simulink model "can_decoder"  (R2025a)
settings: configuration reference "AMCBLDC_Configuration" (kept outside this file)
undefined symbols (not defined in the file): CAN_ID_AMC, CAN_VOLT_REF_GAIN, CAN_VOLT_REF_SHIFT
settings Model: DataDictionary=amcbldc.sldd  Creator=upattacini  LastModifiedBy=rpumpo
settings ConfigSetRef: SourceName=AMCBLDC_Configuration

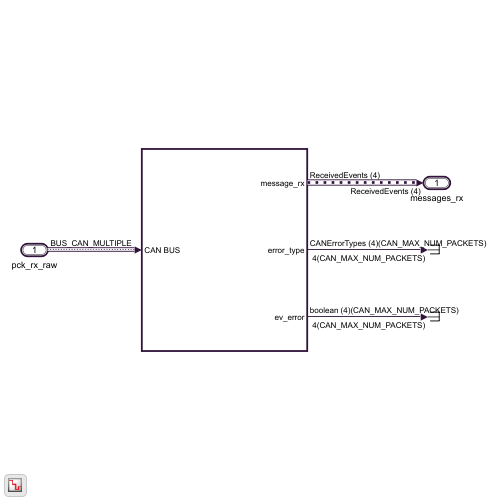
[thumbnail: Simulink's stored preview of the top-level diagram]
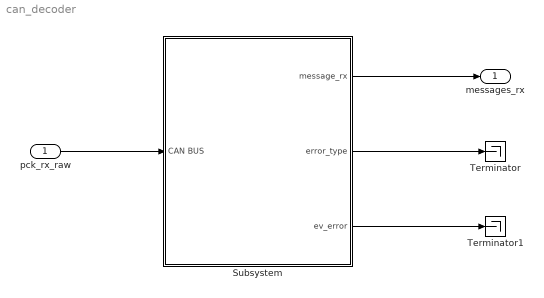
== system can_decoder ==
  pck_rx_raw : Inport  OutDataTypeStr=Bus: BUS_CAN_MULTIPLE  BusOutputAsStruct=on
  Subsystem : Subsystem
  Terminator : Terminator
  Terminator1 : Terminator
  messages_rx : Outport  OutDataTypeStr=Bus: ReceivedEvents  BusOutputAsStruct=on
  wires:
  pck_rx_raw/1 -> Subsystem/1(CAN BUS)
  Subsystem/1(message_rx) -> messages_rx/1
  Subsystem/2(error_type) -> Terminator/1
  Subsystem/3(ev_error) -> Terminator1/1

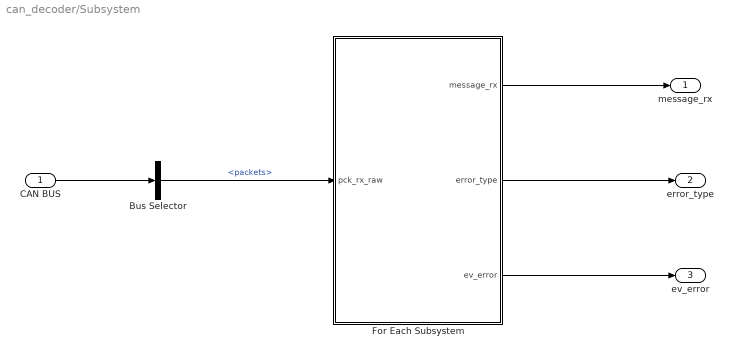
== system can_decoder/Subsystem ==
  CAN BUS : Inport
  Bus Selector : BusSelector  OutputSignals=packets
  For Each Subsystem : Subsystem  TreatAsAtomicUnit=on
  message_rx : Outport  PortDimensions=4
  error_type : Outport  Port=2
  ev_error : Outport  Port=3
  wires:
  Bus Selector/1 -> For Each Subsystem/1(pck_rx_raw)  "<packets>"
  CAN BUS/1 -> Bus Selector/1
  For Each Subsystem/3(ev_error) -> ev_error/1
  For Each Subsystem/1(message_rx) -> message_rx/1
  For Each Subsystem/2(error_type) -> error_type/1

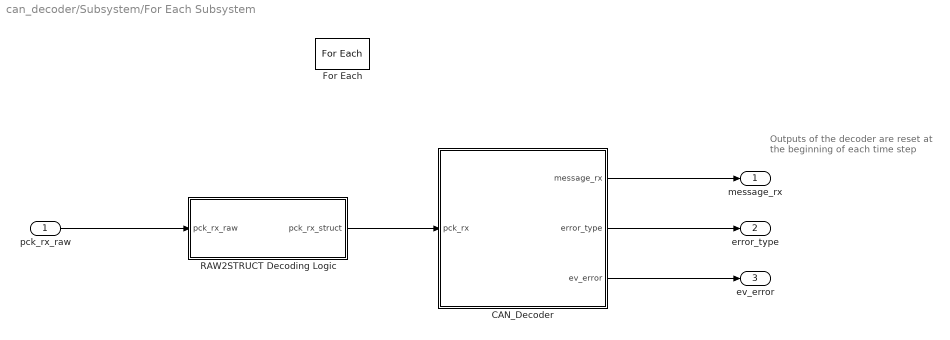
== system can_decoder/Subsystem/For Each Subsystem ==
  note: Outputs of the decoder are reset at
      | the beginning of each time step
  pck_rx_raw : Inport  Partition=on  PartitionDimension=1  PartitionWidth=1  PartitionOffset=0
  CAN_Decoder : Subsystem  TreatAsAtomicUnit=on
  For Each : ForEach  DisableCoverage=on  SpecifiedNumIters=CAN_MAX_NUM_PACKETS
  RAW2STRUCT Decoding Logic : MATLAB Function  TreatAsAtomicUnit=on
  message_rx : Outport  OutDataTypeStr=Bus: ReceivedEvents  ConcatenationDimension=1
  error_type : Outport  Port=2  ConcatenationDimension=1
  ev_error : Outport  Port=3  ConcatenationDimension=1
  wires:
  CAN_Decoder/3(ev_error) -> ev_error/1
  RAW2STRUCT Decoding Logic/1(pck_rx_struct) -> CAN_Decoder/1(pck_rx)
  CAN_Decoder/1(message_rx) -> message_rx/1
  pck_rx_raw/1 -> RAW2STRUCT Decoding Logic/1(pck_rx_raw)
  CAN_Decoder/2(error_type) -> error_type/1

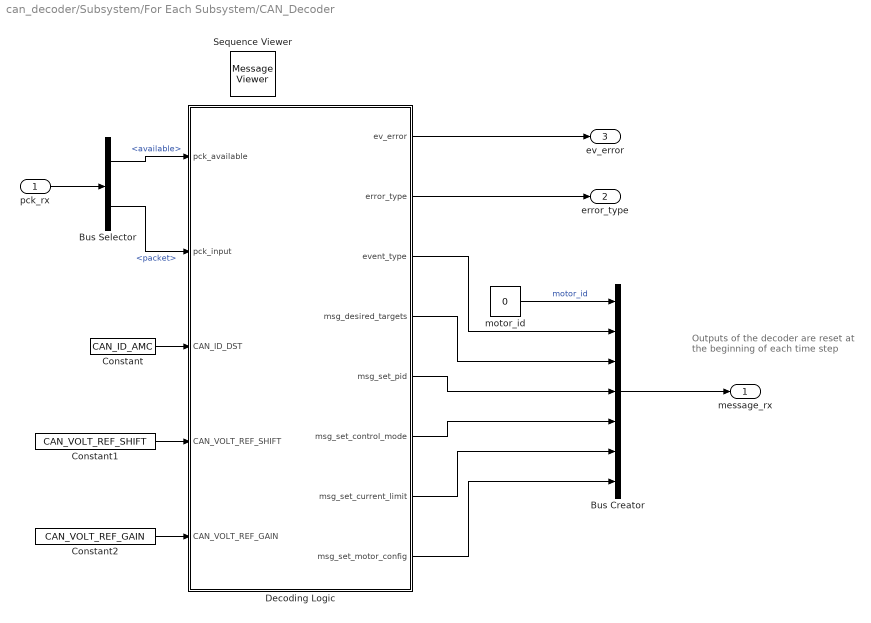
== system can_decoder/Subsystem/For Each Subsystem/CAN_Decoder ==
  note: Outputs of the decoder are reset at
      | the beginning of each time step
  pck_rx : Inport  OutDataTypeStr=Bus: BUS_CAN_RX
  Bus Creator : BusCreator  Inputs=7  OutDataTypeStr=Bus: ReceivedEvents  NonVirtualBus=on
      settings: InheritFromInputs=off
  Bus Selector : BusSelector  OutputSignals=available,packet
  Constant : Constant  Value=CAN_ID_AMC  OutDataTypeStr=uint8
  Constant1 : Constant  Value=CAN_VOLT_REF_SHIFT  OutDataTypeStr=uint8
  Constant2 : Constant  Value=CAN_VOLT_REF_GAIN  OutDataTypeStr=single
  Decoding Logic : Stateflow chart  TreatAsAtomicUnit=on
      settings: PortSchema="{\"entries\":[{\"content\":{\"sides\":[{\"content\":{\"connectorIds\":[\"In1\",\"In2\",\"In3\",\"In4\",\"In5\"]},\"type\":\"ConnectorPlacement.EquallySpacedRectSide\",\"uuid\":\"bb5ffdcb-390f-4d7b-9f99-b75bae8a05ad\"},{\"content\":{\"connectorIds\":[\"Out8\",\"Out6\",\"Out7\",\"Out3\",\"Out4\",\"Out1\",\"Out2\",\"Out5\"],\"side\":\"RIGHT\"},\"type\":\"ConnectorPlacement.EquallySpacedRectSide\",\"uuid\":\"3ba90815-a3e4-4cd4-b64a-5c95e1f5d631\"},{\"content\":{\"side\":\"TOP\"},\"type\":\"ConnectorPlacement.EquallySpacedRectSide\",\"uuid\":\"c9c9b262-1031-4ca9-8b93-619604387376\"}]},\"type\":\"ConnectorPlacement.EquallySpacedConnector\",\"uuid\":\"025015ea-955c-40a8-a93e-b34368e10f0a\"}],\"packageUris\":[\"http://schema.mathworks.com/mf0/Connector/R2020b\"],\"version\":\"1.0\"}"
  Sequence Viewer : MessageViewer
  motor_id : Constant  Value=0  OutDataTypeStr=uint8
  message_rx : Outport  OutDataTypeStr=Bus: ReceivedEvents
  error_type : Outport  Port=2
  ev_error : Outport  Port=3
  wires:
  Constant/1 -> Decoding Logic/3(CAN_ID_DST)
  pck_rx/1 -> Bus Selector/1
  Bus Selector/1 -> Decoding Logic/1(pck_available)  "<available>"
  Bus Selector/2 -> Decoding Logic/2(pck_input)  "<packet>"
  Constant1/1 -> Decoding Logic/4(CAN_VOLT_REF_SHIFT)
  Constant2/1 -> Decoding Logic/5(CAN_VOLT_REF_GAIN)
  Decoding Logic/8(ev_error) -> ev_error/1
  Decoding Logic/6(error_type) -> error_type/1
  Bus Creator/1 -> message_rx/1
  Decoding Logic/7(event_type) -> Bus Creator/2
  Decoding Logic/3(msg_desired_targets) -> Bus Creator/3
  Decoding Logic/4(msg_set_pid) -> Bus Creator/4
  Decoding Logic/1(msg_set_control_mode) -> Bus Creator/5
  Decoding Logic/2(msg_set_current_limit) -> Bus Creator/6
  Decoding Logic/5(msg_set_motor_config) -> Bus Creator/7
  motor_id/1 -> Bus Creator/1  "motor_id"

== stateflow chart can_decoder/Subsystem/For Each Subsystem/CAN_Decoder/Decoding Logic ==
  settings: initializeOutput=1  description=This state chart is responsible for decoding incoming CAN packets.
  state ErrorHandler [parallel]
    settings: executionOrder=2
    state Home
      entry:
      cmd_processed = 0;
      exit:
      ev_async = false;
    state Event_Error
      entry:
      ev_async = true;
    (default) -> ErrorHandler.Home
    (junction 111) -> ErrorHandler.Home [order 2] : {error_type = CANErrorTypes.No_Error;}
    (junction 111) -> ErrorHandler.Home [order 1] : [cmd_processed > 1]
        | {error_type = CANErrorTypes.Packet_MultiFunctionsDetected;
        | send(ev_error);}
    ErrorHandler.Home -> ErrorHandler.Home [order 4] : [ev_async]
    (junction 109) -> ErrorHandler.Home [order 1] : [pck_available && (cmd_processed == 0)]
        | {error_type = CANErrorTypes.Packet_Unrecognized;
        | send(ev_error);}
    Event_Error -> ErrorHandler.Home
    ErrorHandler.Home -> Event_Error [order 1] : ev_error_pck_not4us
        | {error_type = CANErrorTypes.Packet_Not4Us;
        | send(ev_error);}
    ErrorHandler.Home -> Event_Error [order 2] : ev_error_pck_malformed
        | {error_type = CANErrorTypes.Packet_Malformed;
        | send(ev_error);}
    ErrorHandler.Home -> Event_Error [order 3] : ev_error_mode_unrecognized
        | {error_type = CANErrorTypes.Mode_Unrecognized;
        | send(ev_error);}
    ErrorHandler.Home -> (junction 109) [order 5]
    (junction 109) -> (junction 111) [order 2]
  state CANParser [parallel]
    settings: executionOrder=1
    state Home
    state SetCommand [function]
      state r = isPayloadValid(expected_size) [function]
        (default) -> (junction 402) : {r = true;}
        (junction 402) -> (junction 503) [order 1] : [pck_input.ID.DST_TYP != CAN_ID_DST]{send(ev_error_pck_not4us, ErrorHandler); r = false;}
        (junction 402) -> (junction 505) [order 2] : [pck_input.PAYLOAD.LEN < 1]{send(ev_error_pck_malformed, ErrorHandler); r = false;}
        (junction 402) -> (junction 507) [order 3] : [pck_input.PAYLOAD.LEN <  expected_size]
            | {send(ev_error_pck_malformed, ErrorHandler);; r = false;}
      state SetControlMode [function]
        (default) -> (junction 510)
        (junction 510) -> (junction 339) [order 2] : {mc_mode =  pck_input.PAYLOAD.ARG[1];}
        (junction 339) -> (junction 406) [order 2] : {% msg_set_control_mode.motor = pck_input.PAYLOAD.CMD.M;
            | msg_set_control_mode = convertMode(mc_mode);
            | cmd_processed++;
            | event_type = EventTypes.SetControlMode;}
        (junction 510) -> (junction 523) [order 1] : [!isPayloadValid(2)]
        (junction 339) -> (junction 408) [order 1] : [!is_controlmode_recognized(mc_mode)]
            | {send(ev_error_mode_unrecognized, ErrorHandler);}
      state SetCurrentLimits [function]
        (default) -> (junction 381)
        (junction 381) -> (junction 527) [order 1] : [!isPayloadValid(8)]
        (junction 381) -> (junction 382) [order 2] : {% msg_set_current_limit.motor = pck_input.PAYLOAD.CMD.M;
            | msg_set_current_limit.nominal = single(0.001)*single(merge_2bytes_signed(pck_input.PAYLOAD.ARG[2], pck_input.PAYLOAD.ARG[3]));
            | msg_set_current_limit.peak = single(0.001)*single(merge_2bytes_unsigned(pck_input.PAYLOAD.ARG[4], pck_input.PAYLOAD.ARG[5]));
            | msg_set_current_limit.overload = single(0.001)*single(merge_2bytes_unsigned(pck_input.PAYLOAD.ARG[6], pck_input.PAYLOAD.ARG[7]));
            | cmd_processed++;
            | event_type = EventTypes.SetLimit;}
      state SetMotorConfig [function]
        (default) -> (junction 397)
        (junction 397) -> (junction 530) [order 1] : [!isPayloadValid(8)]
        (junction 397) -> (junction 398) [order 2] : {msg_set_motor_config.has_quadrature_encoder = boolean(pck_input.PAYLOAD.ARG[1] & 0x01);
            | msg_set_motor_config.has_hall_sens = boolean(pck_input.PAYLOAD.ARG[1] & 0x02);
            | msg_set_motor_config.has_temperature_sens = boolean(pck_input.PAYLOAD.ARG[1] & 0x04);
            | msg_set_motor_config.use_index = boolean(pck_input.PAYLOAD.ARG[1] & 0x08);
            | msg_set_motor_config.has_speed_quadrature_encoder = boolean(pck_input.PAYLOAD.ARG[1] & 0x10);
            | msg_set_motor_config.enable_verbosity = boolean(pck_input.PAYLOAD.ARG[1] & 0x20);
            | msg_set_motor_config.rotor_encoder_resolution = merge_2bytes_signed(pck_input.PAYLOAD.ARG[2], pck_input.PAYLOAD.ARG[3]);
            | msg_set_motor_config.rotor_index_offset = merge_2bytes_signed(pck_input.PAYLOAD.ARG[4], pck_input.PAYLOAD.ARG[5]);
            | msg_set_motor_config.pole_pairs = pck_input.PAYLOAD.ARG[6] / 2;
            | msg_set_motor_config.encoder_tolerance = pck_input.PAYLOAD.ARG[7];
            | cmd_processed++;
            | event_type = EventTypes.SetMotorConfig;}
      state SetCurrentPID [function]
        (default) -> (junction 386)
        (junction 386) -> (junction 532) [order 1] : [!isPayloadValid(8)]
        (junction 386) -> (junction 387) [order 2] : {%msg_set_pid.motor = pck_input.PAYLOAD.CMD.M;
            | msg_set_pid.shift_factor = pck_input.PAYLOAD.ARG[7];
            | c = single(0x01 << (15 - msg_set_pid.shift_factor)) / single(32768);
            | msg_set_pid.P = c * single(merge_2bytes_signed(pck_input.PAYLOAD.ARG[1], pck_input.PAYLOAD.ARG[2]));
            | msg_set_pid.I = c * single(merge_2bytes_signed(pck_input.PAYLOAD.ARG[3], pck_input.PAYLOAD.ARG[4]));
            | msg_set_pid.D = c * single(merge_2bytes_signed(pck_input.PAYLOAD.ARG[5], pck_input.PAYLOAD.ARG[6]));
            | msg_set_pid.type = ControlModes.Current;
            | cmd_processed++;}
      state SetVelocityPID [function]
        (default) -> (junction 391)
        (junction 391) -> (junction 534) [order 1] : [!isPayloadValid(8)]
        (junction 391) -> (junction 392) [order 2] : {msg_set_pid.shift_factor = pck_input.PAYLOAD.ARG[7];
            | c = single(0x01 << (15 - msg_set_pid.shift_factor)) / single(32768);
            | msg_set_pid.P = c * single(merge_2bytes_signed(pck_input.PAYLOAD.ARG[1], pck_input.PAYLOAD.ARG[2]));
            | msg_set_pid.I = c * single(merge_2bytes_signed(pck_input.PAYLOAD.ARG[3], pck_input.PAYLOAD.ARG[4]));
            | msg_set_pid.D = c * single(merge_2bytes_signed(pck_input.PAYLOAD.ARG[5], pck_input.PAYLOAD.ARG[6]));
            | msg_set_pid.P *= single(0.001);
            | msg_set_pid.I *= single(0.001);
            | msg_set_pid.D *= single(0.001);
            | msg_set_pid.type = ControlModes.Velocity;
            | event_type = EventTypes.SetPid;}
      state SetPositionPID [function]
        (default) -> (junction 601)
        (junction 601) -> (junction 602) [order 2] : {msg_set_pid.shift_factor = pck_input.PAYLOAD.ARG[7];
            | c = single(0x01 << (15 - msg_set_pid.shift_factor)) / single(32768);
            | msg_set_pid.P = c * single(merge_2bytes_signed(pck_input.PAYLOAD.ARG[1], pck_input.PAYLOAD.ARG[2]));
            | msg_set_pid.I = c * single(merge_2bytes_signed(pck_input.PAYLOAD.ARG[3], pck_input.PAYLOAD.ARG[4]));
            | msg_set_pid.D = c * single(merge_2bytes_signed(pck_input.PAYLOAD.ARG[5], pck_input.PAYLOAD.ARG[6]));
            | msg_set_pid.type = ControlModes.Position;
            | event_type = EventTypes.SetPid;}
        (junction 601) -> (junction 600) [order 1] : [!isPayloadValid(8)]
      (default) -> (junction 310)
      (junction 310) -> (junction 587) [order 1] : [pck_input.PAYLOAD.CMD.OPC == MCOPC.Set_Control_Mode]
      (junction 587) -> (junction 312) : {SetControlMode();}
      (junction 310) -> (junction 314) [order 2]
      (junction 312) -> (junction 316)
      (junction 314) -> (junction 585) [order 1] : [pck_input.PAYLOAD.CMD.OPC == MCOPC.Set_Current_Limit]
      (junction 585) -> (junction 316) : {SetCurrentLimits();}
      (junction 314) -> (junction 318) [order 2]
      (junction 316) -> (junction 321)
      (junction 318) -> (junction 583) [order 1] : [pck_input.PAYLOAD.CMD.OPC == MCOPC.Set_Motor_Config]
      (junction 583) -> (junction 321) : {SetMotorConfig();}
      (junction 318) -> (junction 324) [order 2]
      (junction 321) -> (junction 322)
      (junction 324) -> (junction 581) [order 1] : [pck_input.PAYLOAD.CMD.OPC == MCOPC.Set_Current_PID]
      (junction 581) -> (junction 322) : {SetCurrentPID();}
      (junction 324) -> (junction 328) [order 2]
      (junction 322) -> (junction 326)
      (junction 328) -> (junction 589) [order 1] : [pck_input.PAYLOAD.CMD.OPC == MCOPC.Set_Velocity_PID]
      (junction 589) -> (junction 326) : {SetVelocityPID();}
      (junction 328) -> (junction 607) [order 2]
      (junction 326) -> (junction 611)
      (junction 607) -> (junction 606) [order 1] : [pck_input.PAYLOAD.CMD.OPC == MCOPC.Set_Position_PID]
      (junction 606) -> (junction 611) : {SetPositionPID();}
      (junction 607) -> (junction 334) [order 2]
      (junction 611) -> (junction 576)
      (junction 576) -> (junction 334)
      (junction 334) -> (junction 579) : //default
    state SetStreaming [function]
      state SetTargets [function]
        (default) -> (junction 372)
        (junction 372) -> (junction 373) : [(pck_input.PAYLOAD.LEN == 8) && (CAN_ID_DST <= 4)]
            | {idx = 2*(CAN_ID_DST-1);
            |  idx_time = 2*(CAN_ID_DST);
            | tmp_merged = merge_2bytes_signed(pck_input.PAYLOAD.ARG[idx], pck_input.PAYLOAD.ARG[idx+1]);
            | tmp_time = merge_2bytes_signed(pck_input.PAYLOAD.ARG[idx_time], pck_input.PAYLOAD.ARG[idx_time+1]);
            | msg_desired_targets.current = single(0.001) * single(tmp_merged);
            | msg_desired_targets.voltage = single(tmp_merged >> CAN_VOLT_REF_SHIFT) / CAN_VOLT_REF_GAIN;
            | msg_desired_targets.velocity = single(1000) * single(tmp_merged) * CAN_ANGLE_ICUB2DEG;
            | msg_desired_targets.position = single(1000) * single(tmp_merged) * CAN_ANGLE_ICUB2DEG;
            | msg_desired_targets.trajectory_time = single(0.5);
            | cmd_processed++;
            | event_type = EventTypes.SetTarget;}
      (default) -> (junction 344)
      (junction 344) -> (junction 345) : [ (MCStreaming(pck_input.ID.DST_TYP) == MCStreaming.Desired_Targets)]
          | {SetTargets();}
    (default) -> CANParser.Home
    CANParser.Home -> (junction 535) : [pck_available]
    (junction 535) -> (junction 303) [order 1] : [(pck_input.ID.CLS == CANClassTypes.Motor_Control_Command)]
        | {SetCommand();}
    (junction 535) -> CANParser.Home [order 3]
    (junction 535) -> (junction 303) [order 2] : [(pck_input.ID.CLS == CANClassTypes.Motor_Control_Streaming)]
        | {SetStreaming();}
    (junction 303) -> CANParser.Home
  data: ev_async local boolean =false; expected_size function_input uint8; r function_output boolean; MCMode function_input Enum: MCControlModes; mode function_output Enum: ControlModes; mode function_input int32; ok function_output boolean; bl function_input uint16; bh function_input uint16; uw function_output uint16; bl function_input uint16; bh function_input uint16; sw function_output int16; pck_available input boolean; pck_input input Bus: BUS_CAN_PACKET_RX; CAN_ID_DST input uint8; msg_set_control_mode output Enum: ControlModes; msg_set_current_limit output Bus: SupervisorInputLimits; msg_desired_targets output Bus: Targets; msg_set_pid output Bus: PID; msg_set_motor_config output Bus: MotorConfigurationExternal; error_type output Enum: CANErrorTypes size=1 =CANErrorTypes.No_Error; cmd_processed local uint16 size=1 =0; CAN_VOLT_REF_SHIFT input uint8; CAN_VOLT_REF_GAIN input single; CAN_ANGLE_ICUB2DEG parameter; event_type output Enum: EventTypes =EventTypes.None; c local double; tmp_merged local double; idx local double; mc_mode local double; idx_time local double; tmp_time local double
  data CAN_ID_DST settings: description=The ID of the receiver.
  data msg_set_control_mode settings: description=Contains the data to set the required control mode.
  data msg_set_current_limit settings: description=Contains the data to set the required current limit.
  data msg_desired_targets settings: description=Contains the data to set the required current limit.
  data msg_set_pid settings: description=Contains the data to set the required current limit.
  data msg_set_motor_config settings: description=Contains the data to set the required current limit.
  events: ev_error_mode_unrecognized local FUNCTION_CALL_EVENT; ev_error output EITHER_EDGE_EVENT; ev_error_pck_malformed local FUNCTION_CALL_EVENT; ev_error_pck_not4us local FUNCTION_CALL_EVENT
  function mode = convertMode(MCMode):
    | function mode = convertMode(MCMode)
    | 
    |     if MCMode == MCControlModes.Idle
    |         mode = ControlModes.Idle;
    |     elseif MCMode == MCControlModes.Current
    |         mode = ControlModes.Current;
    |     elseif MCMode == MCControlModes.SpeedVoltage
    |         mode = ControlModes.Velocity;
    |     elseif MCMode == MCControlModes.OpenLoop
    |         mode = ControlModes.Voltage;
    |     elseif MCMode == MCControlModes.Position
    |         mode = ControlModes.Position;
    |     else
    |         mode = ControlModes.Idle;
    |     end
    | 
    | end
  function ok = is_controlmode_recognized(mode):
    | function ok = is_controlmode_recognized(mode) 
    | 
    | ok = true;
    | if (mode ~= MCControlModes.Idle)         && ...
    |    (mode ~= MCControlModes.OpenLoop)     && ...
    |    (mode ~= MCControlModes.SpeedVoltage) && ...
    |    (mode ~= MCControlModes.Current)      && ...
    |    (mode ~= MCControlModes.Position)
    |     ok = false;
    | end
  function uw = merge_2bytes_unsigned(bl, bh):
    | function uw = merge_2bytes_unsigned(bl, bh)
    | 
    | uw = bitor(bitshift(bh, 8), bl);
  function sw = merge_2bytes_signed(bl, bh):
    | function sw = merge_2bytes_signed(bl, bh)
    | 
    | uw = bitor(bitshift(bh, 8), bl);
    | sw = typecast(uw, 'int16');

== matlab function can_decoder/Subsystem/For Each Subsystem/RAW2STRUCT Decoding Logic ==
  data: pck_rx_raw input Bus: BUS_CAN; pck_rx_struct output Bus: BUS_CAN_RX
function pck_rx_struct = raw2struct(pck_rx_raw)

pck_rx_struct.available = pck_rx_raw.available;

% ID
pck_rx_struct.packet.ID.CLS = CANClassTypes(bitshift(bitand(pck_rx_raw.packet.ID, 0x0700), -8));
pck_rx_struct.packet.ID.SRC = uint8(bitshift(bitand(pck_rx_raw.packet.ID, 0x0f0), -4));
pck_rx_struct.packet.ID.DST_TYP = uint8(bitand(pck_rx_raw.packet.ID, 0x00f));

% PAYLOAD
pck_rx_struct.packet.PAYLOAD.LEN = max([0, min([8, pck_rx_raw.length])]);
pck_rx_struct.packet.PAYLOAD.CMD.M = (bitand(pck_rx_raw.packet.PAYLOAD(1), 0x80) ~= 0);
pck_rx_struct.packet.PAYLOAD.CMD.OPC = bitand(pck_rx_raw.packet.PAYLOAD(1), 0x7f);

% We get both the polling and the streaming packtes covered
pck_rx_struct.packet.PAYLOAD.ARG = pck_rx_raw.packet.PAYLOAD;
